simulink model "alocacao_polos"  (R2018a)
settings: Solver=VariableStepAuto  StartTime=0.0  StopTime=100  RelTol=1e-3
undefined symbols (not defined in the file): k, ki, model_tf4, x0_tf4
settings Model: Creator=Usuario  LastModifiedBy=Usuario

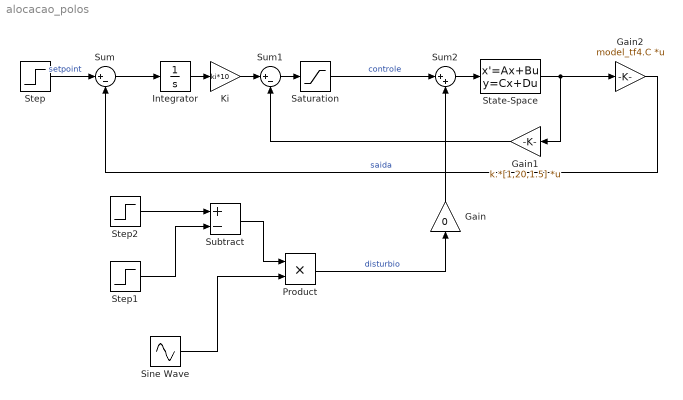
== system alocacao_polos ==
  Gain : Gain  Gain=0
  Gain1 : Gain  Gain=k.*[1,20,1.5]  Multiplication=Matrix(K*u)
  Gain2 : Gain  Gain=model_tf4.C  Multiplication=Matrix(K*u)
  Integrator : Integrator
  Ki : Gain  Gain=ki*10
  Product : Product
  Saturation : Saturate  UpperLimit=254  LowerLimit=0  OutMin=0  OutMax=254
  Sine Wave : Sin  Amplitude=10  SampleTime=0
  State-Space : StateSpace  A=model_tf4.A  B=model_tf4.B  C=eye(3)  D=[0;0;0]  InitialCondition=x0_tf4
  Step : Step  Time=100  Before=70  After=70  SampleTime=0.05
  Step1 : Step  Time=30  Before=10  After=10  SampleTime=0.05
  Step2 : Step  Time=100  Before=10  After=10  SampleTime=0.05
  Subtract : Sum  Inputs=+-
  Sum : Sum  Inputs=|+-
  Sum1 : Sum  Inputs=|+-
  Sum2 : Sum  Inputs=|++
  wires:
  Sum2/1 -> State-Space/1
  State-Space/1 -> Gain2/1, Gain1/1
  Gain1/1 -> Sum1/2
  Step2/1 -> Subtract/1
  Step1/1 -> Subtract/2
  Sine Wave/1 -> Product/2
  Subtract/1 -> Product/1
  Product/1 -> Gain/1  "disturbio"
  Gain2/1 -> Sum/2  "saida"
  Gain/1 -> Sum2/2
  Integrator/1 -> Ki/1
  Ki/1 -> Sum1/1
  Sum/1 -> Integrator/1
  Step/1 -> Sum/1  "setpoint"
  Saturation/1 -> Sum2/1  "controle"
  Sum1/1 -> Saturation/1
